simulink model "logic_operations_with_switch"  (R2017b)
settings: Solver=FixedStepDiscrete  StartTime=0.0  StopTime=10.0  RelTol=1e-3
settings Model: Creator=ebrah  LastModifiedBy=ebrah
settings OptimizationCC: DefaultParameterBehavior=Inlined  PassReuseOutputArgsAs=Individual arguments
settings DebuggingCC: ParameterTunabilityLossMsg=error
settings SFSimCC: MATLABDynamicMemAlloc=off
settings RTWCC: SystemTargetFile=ert.tlc  GenCodeOnly=on  TemplateMakefile=ert_default_tmf  GenerateReport=on  IncludeHyperlinkInReport=on  LaunchReport=on  GenerateTraceInfo=on  GenerateTraceReport=on  GenerateTraceReportSl=on  GenerateTraceReportSf=on  GenerateTraceReportEml=on  GenerateWebview=on
settings CodeAppCC: ForceParamTrailComments=on  IgnoreCustomStorageClasses=off  OperatorAnnotations=on  SimulinkDataObjDesc=on  SFDataObjDesc=on  InsertBlockDesc=on
settings ERTTargetCC: TargetLangStandard=C99 (ISO)  GenerateSampleERTMain=on  InlinedParameterPlacement=NonHierarchical  ERTCustomFileTemplate=example_file_process.tlc

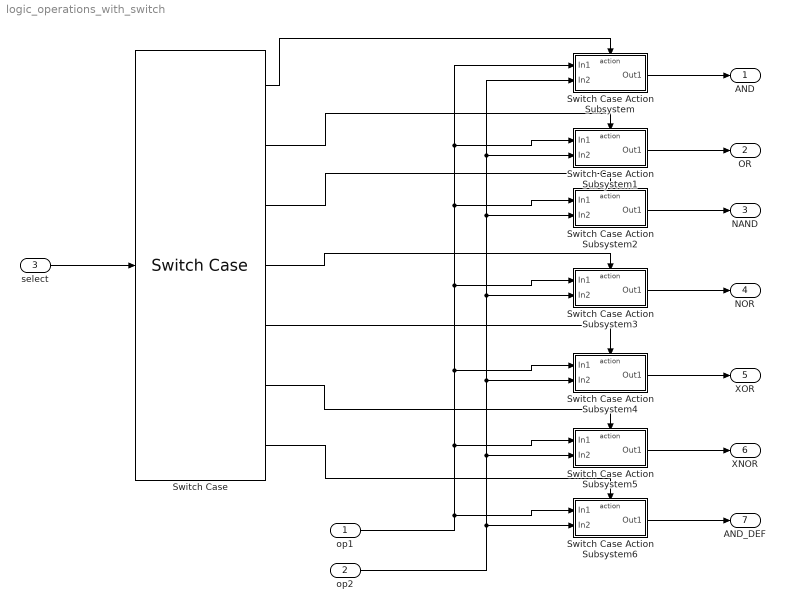
== system logic_operations_with_switch ==
  op1 : Inport
  op2 : Inport  Port=2
  select : Inport  Port=3
  Switch Case : SwitchCase  CaseConditions={1,2,3,4,5, 6}
  Switch Case Action Subsystem : Subsystem  TreatAsAtomicUnit=on
  Switch Case Action Subsystem1 : Subsystem  TreatAsAtomicUnit=on
  Switch Case Action Subsystem2 : Subsystem  TreatAsAtomicUnit=on
  Switch Case Action Subsystem3 : Subsystem  TreatAsAtomicUnit=on
  Switch Case Action Subsystem4 : Subsystem  TreatAsAtomicUnit=on
  Switch Case Action Subsystem5 : Subsystem  TreatAsAtomicUnit=on
  Switch Case Action Subsystem6 : Subsystem  TreatAsAtomicUnit=on
  AND : Outport
  OR : Outport  Port=2
  NAND : Outport  Port=3
  NOR : Outport  Port=4
  XOR : Outport  Port=5
  XNOR : Outport  Port=6
  AND_DEF : Outport  Port=7
  wires:
  Switch Case/1 -> Switch Case Action Subsystem/Action
  Switch Case/2 -> Switch Case Action Subsystem1/Action
  Switch Case/3 -> Switch Case Action Subsystem2/Action
  Switch Case/4 -> Switch Case Action Subsystem3/Action
  Switch Case/5 -> Switch Case Action Subsystem4/Action
  Switch Case/6 -> Switch Case Action Subsystem5/Action
  Switch Case/7 -> Switch Case Action Subsystem6/Action
  op1/1 -> Switch Case Action Subsystem6/1(In1), Switch Case Action Subsystem5/1(In1), Switch Case Action Subsystem4/1(In1), Switch Case Action Subsystem3/1(In1), Switch Case Action Subsystem2/1(In1), Switch Case Action Subsystem1/1(In1), Switch Case Action Subsystem/1(In1)
  op2/1 -> Switch Case Action Subsystem6/2(In2), Switch Case Action Subsystem5/2(In2), Switch Case Action Subsystem4/2(In2), Switch Case Action Subsystem3/2(In2), Switch Case Action Subsystem2/2(In2), Switch Case Action Subsystem1/2(In2), Switch Case Action Subsystem/2(In2)
  select/1 -> Switch Case/1
  Switch Case Action Subsystem/1(Out1) -> AND/1
  Switch Case Action Subsystem1/1(Out1) -> OR/1
  Switch Case Action Subsystem2/1(Out1) -> NAND/1
  Switch Case Action Subsystem3/1(Out1) -> NOR/1
  Switch Case Action Subsystem4/1(Out1) -> XOR/1
  Switch Case Action Subsystem5/1(Out1) -> XNOR/1
  Switch Case Action Subsystem6/1(Out1) -> AND_DEF/1

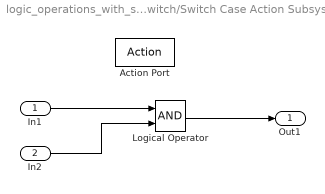
== system logic_operations_with_switch/Switch Case Action Subsystem ==
  In1 : Inport
  In2 : Inport  Port=2
  Action Port : ActionPort  ActionType=case
  Logical Operator : Logic  AllPortsSameDT=off  OutDataTypeStr=boolean
  Out1 : Outport
  wires:
  In1/1 -> Logical Operator/1
  In2/1 -> Logical Operator/2
  Logical Operator/1 -> Out1/1

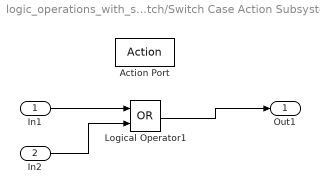
== system logic_operations_with_switch/Switch Case Action Subsystem1 ==
  In1 : Inport
  In2 : Inport  Port=2
  Action Port : ActionPort  ActionType=case
  Logical Operator1 : Logic  Operator=OR  AllPortsSameDT=off  OutDataTypeStr=boolean
  Out1 : Outport
  wires:
  In1/1 -> Logical Operator1/1
  In2/1 -> Logical Operator1/2
  Logical Operator1/1 -> Out1/1

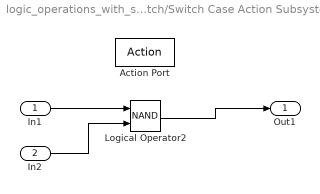
== system logic_operations_with_switch/Switch Case Action Subsystem2 ==
  In1 : Inport
  In2 : Inport  Port=2
  Action Port : ActionPort  ActionType=case
  Logical Operator2 : Logic  Operator=NAND  AllPortsSameDT=off  OutDataTypeStr=boolean
  Out1 : Outport
  wires:
  In1/1 -> Logical Operator2/1
  In2/1 -> Logical Operator2/2
  Logical Operator2/1 -> Out1/1

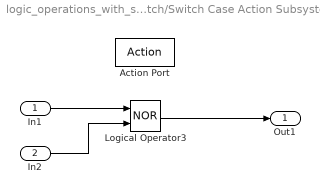
== system logic_operations_with_switch/Switch Case Action Subsystem3 ==
  In1 : Inport
  In2 : Inport  Port=2
  Action Port : ActionPort  ActionType=case
  Logical Operator3 : Logic  Operator=NOR  AllPortsSameDT=off  OutDataTypeStr=boolean
  Out1 : Outport
  wires:
  In1/1 -> Logical Operator3/1
  In2/1 -> Logical Operator3/2
  Logical Operator3/1 -> Out1/1

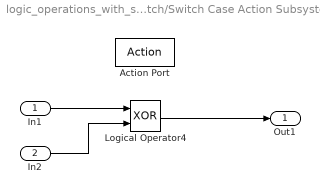
== system logic_operations_with_switch/Switch Case Action Subsystem4 ==
  In1 : Inport
  In2 : Inport  Port=2
  Action Port : ActionPort  ActionType=case
  Logical Operator4 : Logic  Operator=XOR  AllPortsSameDT=off  OutDataTypeStr=boolean
  Out1 : Outport
  wires:
  In1/1 -> Logical Operator4/1
  In2/1 -> Logical Operator4/2
  Logical Operator4/1 -> Out1/1

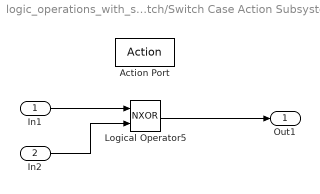
== system logic_operations_with_switch/Switch Case Action Subsystem5 ==
  In1 : Inport
  In2 : Inport  Port=2
  Action Port : ActionPort  ActionType=case
  Logical Operator5 : Logic  Operator=NXOR  AllPortsSameDT=off  OutDataTypeStr=boolean
  Out1 : Outport
  wires:
  In1/1 -> Logical Operator5/1
  In2/1 -> Logical Operator5/2
  Logical Operator5/1 -> Out1/1

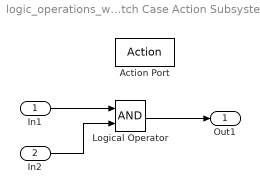
== system logic_operations_with_switch/Switch Case Action Subsystem6 ==
  In1 : Inport
  In2 : Inport  Port=2
  Action Port : ActionPort  ActionType=default
  Logical Operator : Logic  AllPortsSameDT=off  OutDataTypeStr=boolean
  Out1 : Outport
  wires:
  In1/1 -> Logical Operator/1
  In2/1 -> Logical Operator/2
  Logical Operator/1 -> Out1/1
